simulink subsystem "s0518_alpha_theta_PP_int3"  (R2019b)
settings: Solver=VariableStepAuto  StartTime=0.0  StopTime=10.0  RelTol=1e-3
undefined symbols (not defined in the file): __PRM__SERIALIZED__DATA__, den_ref_filter, DiscIntNeverNeededParam, num_ref_filter, PARAMS, SubsystemReferenceBlock
libraries: simulink x1
settings Model: Creator=francescoceresetti  LastModifiedBy=giaco

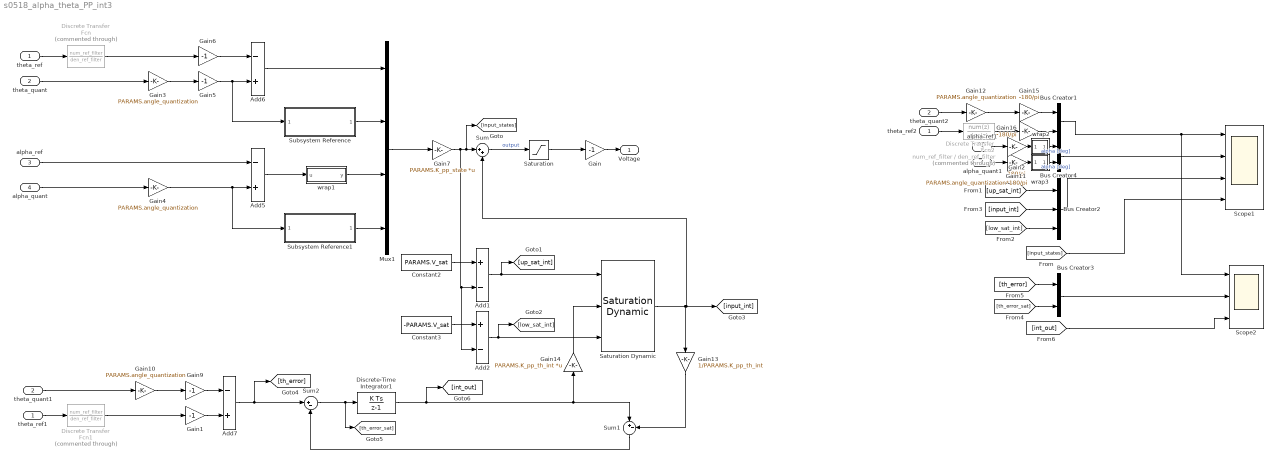
== system s0518_alpha_theta_PP_int3 ==
  theta_ref : Inport
  theta_quant : Inport  Port=2
  alpha_ref : Inport  Port=3
  alpha_quant : Inport  Port=4
  Add1 : Sum  Inputs=+-
  Add2 : Sum  Inputs=+-
  Add5 : Sum  Inputs=-+
  Add6 : Sum  Inputs=-+
  Add7 : Sum  Inputs=-+
  Bus Creator1 : BusCreator  Inputs=2
  Bus Creator2 : BusCreator  Inputs=3
  Bus Creator3 : BusCreator  Inputs=2
  Bus Creator4 : BusCreator  Inputs=2
  Constant2 : Constant  Value=PARAMS.V_sat
  Constant3 : Constant  Value=-PARAMS.V_sat
  Discrete Transfer Fcn : DiscreteTransferFcn  Commented=through  Numerator=num_ref_filter  Denominator=den_ref_filter
  Discrete Transfer Fcn1 : DiscreteTransferFcn  Commented=through  Numerator=num_ref_filter  Denominator=den_ref_filter
  Discrete Transfer Fcn2 : DiscreteTransferFcn  Commented=through  Numerator=num_ref_filter  Denominator=den_ref_filter
  Discrete-Time Integrator1 : DiscreteIntegrator  SampleTime=-1  ICPrevOutput=DiscIntNeverNeededParam  ICPrevScaledInput=DiscIntNeverNeededParam
  Gain{,1,5..6,9} (5 alike) : Gain  Gain=-1
  Gain{3..4,10,12} (4 alike) : Gain  Gain=PARAMS.angle_quantization
  Gain11 : Gain  Gain=PARAMS.angle_quantization*180/pi
  Gain13 : Gain  Gain=1/PARAMS.K_pp_th_int
  Gain14 : Gain  Gain=PARAMS.K_pp_th_int  Multiplication=Matrix(K*u)
  Gain15 : Gain  Gain=-180/pi
  Gain16 : Gain  Gain=-180/pi
  Gain2 : Gain  Gain=180/pi
  Gain7 : Gain  Gain=PARAMS.K_pp_state  Multiplication=Matrix(K*u)
  Mux1 : Mux
  Saturation : Saturate  UpperLimit=PARAMS.V_sat  LowerLimit=-PARAMS.V_sat
  Saturation Dynamic : simulink/Discontinuities/Saturation Dynamic  OutMin=[]  OutMax=[]  OutDataTypeStr=Inherit: Same as second input  OutDataType=fixdt(1, 16)  OutScaling=2^-10  DoSatur=off
  Scope1 : Scope  NumInputPorts=4
  Scope2 : Scope  NumInputPorts=3
  Subsystem Reference : Subsystem  BlockKeywords=__PRM__SERIALIZED__DATA__:SubsystemReferenceBlock  ReferencedSubsystem=Filtered_Derivative  num=num_der_filter  den=den_der_filter
  Subsystem Reference1 : Subsystem  BlockKeywords=__PRM__SERIALIZED__DATA__:SubsystemReferenceBlock  ReferencedSubsystem=Filtered_Derivative  num=num_der_filter  den=den_der_filter
  Sum : Sum  Inputs=|++
  Sum1 : Sum  Inputs=|+-
  Sum2 : Sum  Inputs=|+-
  alpha_quant1 : InportShadow  Port=4
  alpha_ref1 : InportShadow  Port=3
  theta_quant1 : InportShadow  Port=2
  theta_quant2 : InportShadow  Port=2
  theta_ref1 : InportShadow
  theta_ref2 : InportShadow
  wrap1 : MATLAB Function  TreatAsAtomicUnit=on
  wrap2 : MATLAB Function  TreatAsAtomicUnit=on
  wrap3 : MATLAB Function  TreatAsAtomicUnit=on
  Voltage : Outport
  wires:
  Gain3/1 -> Gain5/1
  Mux1/1 -> Gain7/1
  Subsystem Reference1/1 -> Mux1/4
  Gain4/1 -> Add5/2, Subsystem Reference1/1
  Subsystem Reference/1 -> Mux1/2
  Gain5/1 -> Add6/2, Subsystem Reference/1
  alpha_ref/1 -> Add5/1
  Sum/1 -> Saturation/1  "output"
  Add6/1 -> Mux1/1
  Add5/1 -> wrap1/1(u)
  Gain6/1 -> Add6/1
  wrap1/1(y) -> Mux1/3
  theta_quant/1 -> Gain3/1
  theta_ref/1 -> Discrete Transfer Fcn/1
  alpha_quant/1 -> Gain4/1
  Gain1/1 -> Add7/2
  theta_quant1/1 -> Gain10/1
  Gain9/1 -> Add7/1
  Gain10/1 -> Gain9/1
  Saturation Dynamic/1 -> Gain13/1, [input_int], Sum/2
  Discrete-Time Integrator1/1 -> Gain14/1, Sum1/1, [int_out]
  Gain/1 -> Voltage/1
  Saturation/1 -> Gain/1
  Constant2/1 -> Add1/1
  Constant3/1 -> Add2/1
  Add1/1 -> Saturation Dynamic/1, [up_sat_int]
  Add2/1 -> Saturation Dynamic/3, [low_sat_int]
  Sum1/1 -> Sum2/2
  Sum2/1 -> Discrete-Time Integrator1/1, [th_error_sat]
  Add7/1 -> [th_error], Sum2/1
  Gain13/1 -> Sum1/2
  Gain14/1 -> Saturation Dynamic/2
  Discrete Transfer Fcn/1 -> Gain6/1
  theta_ref1/1 -> Discrete Transfer Fcn1/1
  Discrete Transfer Fcn1/1 -> Gain1/1
  Bus Creator2/1 -> Scope1/3
  Bus Creator3/1 -> Scope2/2
  Gain7/1 -> Sum/1, [input_states], Add2/2, Add1/2
  alpha_quant1/1 -> Gain11/1
  Bus Creator4/1 -> Scope1/2
  theta_quant2/1 -> Gain12/1
  Gain12/1 -> Gain15/1
  Gain15/1 -> Bus Creator1/1
  Gain16/1 -> Bus Creator1/2
  Bus Creator1/1 -> Scope1/1, Scope2/1
  [input_states] -> Scope1/4
  [up_sat_int] -> Bus Creator2/1
  [low_sat_int] -> Bus Creator2/3
  [input_int] -> Bus Creator2/2
  [th_error] -> Bus Creator3/1
  [th_error_sat] -> Bus Creator3/2
  [int_out] -> Scope2/3
  theta_ref2/1 -> Discrete Transfer Fcn2/1
  Discrete Transfer Fcn2/1 -> Gain16/1
  wrap2/1(y) -> Bus Creator4/1  "alpha [deg]"
  Gain11/1 -> wrap3/1(u)
  wrap3/1(y) -> Bus Creator4/2  "alpha [deg]"
  alpha_ref1/1 -> Gain2/1
  Gain2/1 -> wrap2/1(u)

== matlab function s0518_alpha_theta_PP_int3/wrap2 ==
  data: u input; y output
function y = wrap(u)
stop_condition = false;
y = u;
while ~stop_condition
    if y > 270
        y = y - 360;
    elseif y < -90
        y = y + 360;
    else
        stop_condition = true;
    end
end

== matlab function s0518_alpha_theta_PP_int3/wrap3 ==
  data: u input; y output
function y = wrap(u)
stop_condition = false;
y = u;
while ~stop_condition
    if y > 270
        y = y - 360;
    elseif y < -90
        y = y + 360;
    else
        stop_condition = true;
    end
end

== matlab function s0518_alpha_theta_PP_int3/wrap1 ==
  data: u input; y output
function y = wrap(u)
stop_condition = false;
y = u;
while ~stop_condition
    if y > pi
        y = y - 2*pi;
    elseif y < -pi
        y = y + 2*pi;
    else
        stop_condition = true;
    end
end
